simulink model "CRTsfun"  (Simulink 8.0)
settings: Solver=ode45  StartTime=0.0  StopTime=10.0  RelTol=1e-3
undefined symbols (not defined in the file or in its folder): vicrt_initcallback, vicrt_initmexcallback, vicrt_inputfile, vicrt_simulationmanager
(part 3 of 3)

== system CRTsfun/VI-CarRealTime/Output_Bus/adapter ==
  inputBus : Inport
  adaBCre : BusCreator  Inputs=24
  adaDemux : Demux  Outputs=24
  adaSel : Selector  InputPortWidth=24  IndexOptions=Select all  Indices=[1 3]  OutputSizes=1
  outputBus : Outport
  wires:
  adaBCre/1 -> outputBus/1
  adaDemux/24 -> adaBCre/24  "aero_forces:yaw_torque"
  adaDemux/23 -> adaBCre/23  "aero_forces:vertical_velocity"
  adaDemux/22 -> adaBCre/22  "aero_forces:steer"
  adaDemux/21 -> adaBCre/21  "aero_forces:side_slip"
  adaDemux/20 -> adaBCre/20  "aero_forces:roll_torque"
  adaDemux/19 -> adaBCre/19  "aero_forces:roll"
  adaDemux/18 -> adaBCre/18  "aero_forces:rear_sideforce"
  adaDemux/17 -> adaBCre/17  "aero_forces:rear_downforce"
  adaDemux/16 -> adaBCre/16  "aero_forces:pitch"
  adaDemux/15 -> adaBCre/15  "aero_forces:longitudinal_velocity"
  adaDemux/14 -> adaBCre/14  "aero_forces:lateral_velocity"
  adaDemux/13 -> adaBCre/13  "aero_forces:height_rear"
  adaDemux/12 -> adaBCre/12  "aero_forces:height_front"
  adaDemux/11 -> adaBCre/11  "aero_forces:height_auxiliary"
  adaDemux/10 -> adaBCre/10  "aero_forces:front_sideforce"
  adaDemux/9 -> adaBCre/9  "aero_forces:front_downforce"
  adaDemux/8 -> adaBCre/8  "aero_forces:drag_torque"
  adaDemux/7 -> adaBCre/7  "aero_forces:drag_force_rear"
  adaDemux/6 -> adaBCre/6  "aero_forces:drag_force_front"
  adaDemux/5 -> adaBCre/5  "aero_forces:drag_force"
  adaDemux/4 -> adaBCre/4  "aero_forces:drag_arm"
  adaDemux/3 -> adaBCre/3  "aero_forces:center_sideforce"
  adaDemux/2 -> adaBCre/2  "aero_forces:center_downforce"
  adaDemux/1 -> adaBCre/1  "aero_forces:aero_balance"
  adaSel/1 -> adaDemux/1
  inputBus/1 -> adaSel/1

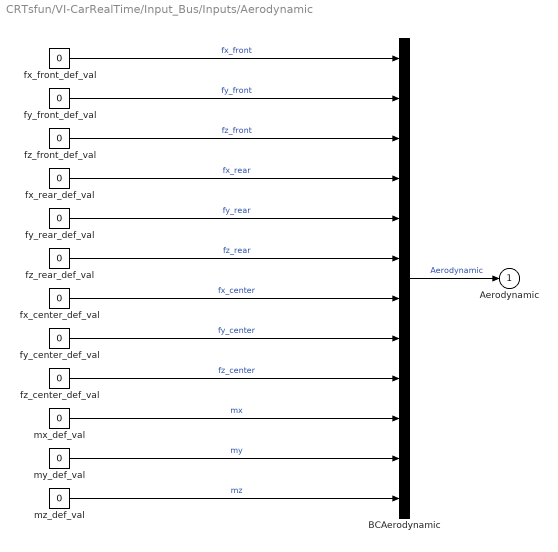
== system CRTsfun/VI-CarRealTime/Input_Bus/Inputs/Aerodynamic ==
  BCAerodynamic : BusCreator  Inputs=12
  fx_center_def_val : Constant  Value=0
  fx_front_def_val : Constant  Value=0
  fx_rear_def_val : Constant  Value=0
  fy_center_def_val : Constant  Value=0
  fy_front_def_val : Constant  Value=0
  fy_rear_def_val : Constant  Value=0
  fz_center_def_val : Constant  Value=0
  fz_front_def_val : Constant  Value=0
  fz_rear_def_val : Constant  Value=0
  mx_def_val : Constant  Value=0
  my_def_val : Constant  Value=0
  mz_def_val : Constant  Value=0
  Aerodynamic : Outport
  wires:
  mz_def_val/1 -> BCAerodynamic/12  "mz"
  my_def_val/1 -> BCAerodynamic/11  "my"
  mx_def_val/1 -> BCAerodynamic/10  "mx"
  fz_center_def_val/1 -> BCAerodynamic/9  "fz_center"
  fy_center_def_val/1 -> BCAerodynamic/8  "fy_center"
  fx_center_def_val/1 -> BCAerodynamic/7  "fx_center"
  fz_rear_def_val/1 -> BCAerodynamic/6  "fz_rear"
  fy_rear_def_val/1 -> BCAerodynamic/5  "fy_rear"
  fx_rear_def_val/1 -> BCAerodynamic/4  "fx_rear"
  fz_front_def_val/1 -> BCAerodynamic/3  "fz_front"
  fy_front_def_val/1 -> BCAerodynamic/2  "fy_front"
  fx_front_def_val/1 -> BCAerodynamic/1  "fx_front"
  BCAerodynamic/1 -> Aerodynamic/1  "Aerodynamic"

== system CRTsfun/VI-CarRealTime/Input_Bus/Inputs/Antiroll_Bar ==
  BCAntiroll_Bar : BusCreator  Inputs=2
  activity_flag : Subsystem
  force : Subsystem
  Antiroll_Bar : Outport
  wires:
  force/1(force) -> BCAntiroll_Bar/2  "force"
  activity_flag/1(activity_flag) -> BCAntiroll_Bar/1  "activity_flag"
  BCAntiroll_Bar/1 -> Antiroll_Bar/1  "Antiroll_Bar"

== system CRTsfun/VI-CarRealTime/Input_Bus/Inputs/Auxiliary_vertical ==
  BCAuxiliary_vertical : BusCreator  Inputs=2
  activity_flag : Subsystem
  force : Subsystem
  Auxiliary_vertical : Outport
  wires:
  activity_flag/1(activity_flag) -> BCAuxiliary_vertical/2  "activity_flag"
  force/1(force) -> BCAuxiliary_vertical/1  "force"
  BCAuxiliary_vertical/1 -> Auxiliary_vertical/1  "Auxiliary_vertical"

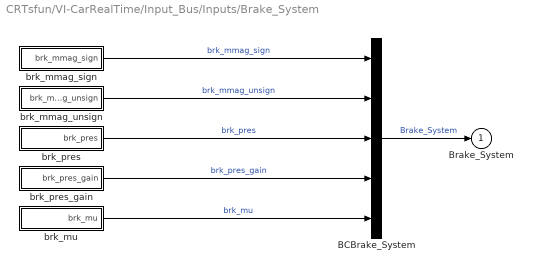
== system CRTsfun/VI-CarRealTime/Input_Bus/Inputs/Brake_System ==
  BCBrake_System : BusCreator  Inputs=5
  brk_mmag_sign : Subsystem
  brk_mmag_unsign : Subsystem
  brk_mu : Subsystem
  brk_pres : Subsystem
  brk_pres_gain : Subsystem
  Brake_System : Outport
  wires:
  brk_mu/1(brk_mu) -> BCBrake_System/5  "brk_mu"
  brk_pres_gain/1(brk_pres_gain) -> BCBrake_System/4  "brk_pres_gain"
  brk_pres/1(brk_pres) -> BCBrake_System/3  "brk_pres"
  brk_mmag_unsign/1(brk_mmag_unsign) -> BCBrake_System/2  "brk_mmag_unsign"
  brk_mmag_sign/1(brk_mmag_sign) -> BCBrake_System/1  "brk_mmag_sign"
  BCBrake_System/1 -> Brake_System/1  "Brake_System"

== system CRTsfun/VI-CarRealTime/Input_Bus/Inputs/Brake_System_General ==
  BCBrake_System_General : BusCreator  Inputs=2
  brk_bias_front_def_val : Constant  Value=0
  brk_mast_cyl_pres_def_val : Constant  Value=0
  Brake_System_General : Outport
  wires:
  brk_bias_front_def_val/1 -> BCBrake_System_General/2  "brk_bias_front"
  brk_mast_cyl_pres_def_val/1 -> BCBrake_System_General/1  "brk_mast_cyl_pres"
  BCBrake_System_General/1 -> Brake_System_General/1  "Brake_System_General"

== system CRTsfun/VI-CarRealTime/Input_Bus/Inputs/Clutch ==
  BCClutch : BusCreator  Inputs=2
  clutch_slip_angle_def_val : Constant  Value=0
  clutch_trq_def_val : Constant  Value=0
  Clutch : Outport
  wires:
  clutch_slip_angle_def_val/1 -> BCClutch/2  "clutch_slip_angle"
  clutch_trq_def_val/1 -> BCClutch/1  "clutch_trq"
  BCClutch/1 -> Clutch/1  "Clutch"

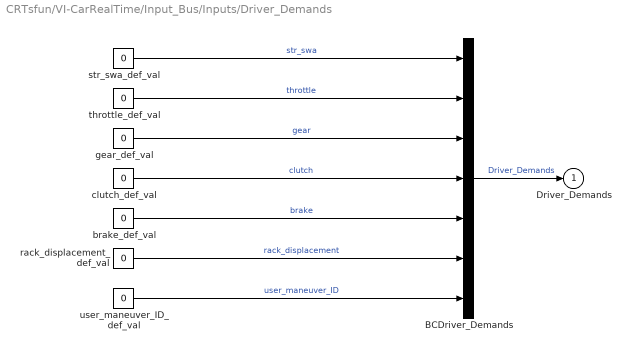
== system CRTsfun/VI-CarRealTime/Input_Bus/Inputs/Driver_Demands ==
  BCDriver_Demands : BusCreator  Inputs=7
  brake_def_val : Constant  Value=0
  clutch_def_val : Constant  Value=0
  gear_def_val : Constant  Value=0
  rack_displacement_def_val : Constant  Value=0
  str_swa_def_val : Constant  Value=0
  throttle_def_val : Constant  Value=0
  user_maneuver_ID_def_val : Constant  Value=0
  Driver_Demands : Outport
  wires:
  user_maneuver_ID_def_val/1 -> BCDriver_Demands/7  "user_maneuver_ID"
  rack_displacement_def_val/1 -> BCDriver_Demands/6  "rack_displacement"
  brake_def_val/1 -> BCDriver_Demands/5  "brake"
  clutch_def_val/1 -> BCDriver_Demands/4  "clutch"
  gear_def_val/1 -> BCDriver_Demands/3  "gear"
  throttle_def_val/1 -> BCDriver_Demands/2  "throttle"
  str_swa_def_val/1 -> BCDriver_Demands/1  "str_swa"
  BCDriver_Demands/1 -> Driver_Demands/1  "Driver_Demands"

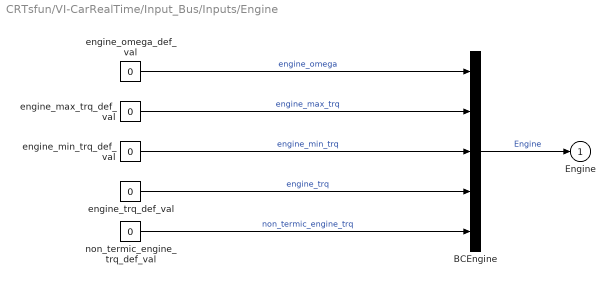
== system CRTsfun/VI-CarRealTime/Input_Bus/Inputs/Engine ==
  BCEngine : BusCreator  Inputs=5
  engine_max_trq_def_val : Constant  Value=0
  engine_min_trq_def_val : Constant  Value=0
  engine_omega_def_val : Constant  Value=0
  engine_trq_def_val : Constant  Value=0
  non_termic_engine_trq_def_val : Constant  Value=0
  Engine : Outport
  wires:
  non_termic_engine_trq_def_val/1 -> BCEngine/5  "non_termic_engine_trq"
  engine_trq_def_val/1 -> BCEngine/4  "engine_trq"
  engine_min_trq_def_val/1 -> BCEngine/3  "engine_min_trq"
  engine_max_trq_def_val/1 -> BCEngine/2  "engine_max_trq"
  engine_omega_def_val/1 -> BCEngine/1  "engine_omega"
  BCEngine/1 -> Engine/1  "Engine"

== system CRTsfun/VI-CarRealTime/Input_Bus/Inputs/Ext_Body ==
  BCExt_Body : BusCreator  Inputs=2
  force : Subsystem
  moment : Subsystem
  Ext_Body : Outport
  wires:
  moment/1(moment) -> BCExt_Body/2  "moment"
  force/1(force) -> BCExt_Body/1  "force"
  BCExt_Body/1 -> Ext_Body/1  "Ext_Body"

== system CRTsfun/VI-CarRealTime/Input_Bus/Inputs/Ext_Ground ==
  BCExt_Ground : BusCreator  Inputs=2
  force : Subsystem
  moment : Subsystem
  Ext_Ground : Outport
  wires:
  moment/1(moment) -> BCExt_Ground/2  "moment"
  force/1(force) -> BCExt_Ground/1  "force"
  BCExt_Ground/1 -> Ext_Ground/1  "Ext_Ground"

== system CRTsfun/VI-CarRealTime/Input_Bus/Inputs/Ext_Tracking ==
  BCExt_Tracking : BusCreator  Inputs=2
  force : Subsystem
  moment : Subsystem
  Ext_Tracking : Outport
  wires:
  moment/1(moment) -> BCExt_Tracking/2  "moment"
  force/1(force) -> BCExt_Tracking/1  "force"
  BCExt_Tracking/1 -> Ext_Tracking/1  "Ext_Tracking"

== system CRTsfun/VI-CarRealTime/Input_Bus/Inputs/Friction ==
  BCFriction : BusCreator  Inputs=1
  tire_mu : Subsystem
  Friction : Outport
  wires:
  tire_mu/1(tire_mu) -> BCFriction/1  "tire_mu"
  BCFriction/1 -> Friction/1  "Friction"

== system CRTsfun/VI-CarRealTime/Input_Bus/Inputs/GearBox ==
  BCGearBox : BusCreator  Inputs=1
  transmission_ratio_def_val : Constant  Value=0
  GearBox : Outport
  wires:
  transmission_ratio_def_val/1 -> BCGearBox/1  "transmission_ratio"
  BCGearBox/1 -> GearBox/1  "GearBox"

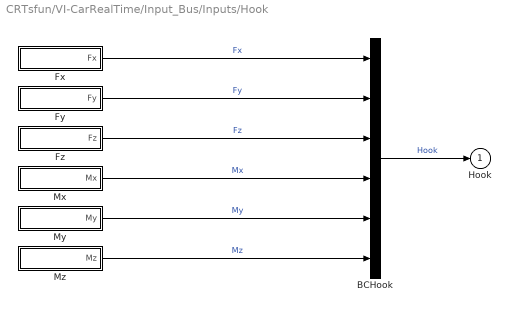
== system CRTsfun/VI-CarRealTime/Input_Bus/Inputs/Hook ==
  BCHook : BusCreator  Inputs=6
  Fx : Subsystem
  Fy : Subsystem
  Fz : Subsystem
  Mx : Subsystem
  My : Subsystem
  Mz : Subsystem
  Hook : Outport
  wires:
  Mz/1(Mz) -> BCHook/6  "Mz"
  My/1(My) -> BCHook/5  "My"
  Mx/1(Mx) -> BCHook/4  "Mx"
  Fz/1(Fz) -> BCHook/3  "Fz"
  Fy/1(Fy) -> BCHook/2  "Fy"
  Fx/1(Fx) -> BCHook/1  "Fx"
  BCHook/1 -> Hook/1  "Hook"

== system CRTsfun/VI-CarRealTime/Input_Bus/Inputs/Irregularity ==
  BCIrregularity : BusCreator  Inputs=1
  road : Subsystem
  Irregularity : Outport
  wires:
  road/1(road) -> BCIrregularity/1  "road"
  BCIrregularity/1 -> Irregularity/1  "Irregularity"

== system CRTsfun/VI-CarRealTime/Input_Bus/Inputs/Main_Bumpstop ==
  BCMain_Bumpstop : BusCreator  Inputs=2
  activity_flag : Subsystem
  force : Subsystem
  Main_Bumpstop : Outport
  wires:
  activity_flag/1(activity_flag) -> BCMain_Bumpstop/2  "activity_flag"
  force/1(force) -> BCMain_Bumpstop/1  "force"
  BCMain_Bumpstop/1 -> Main_Bumpstop/1  "Main_Bumpstop"

== system CRTsfun/VI-CarRealTime/Input_Bus/Inputs/Main_Damper ==
  BCMain_Damper : BusCreator  Inputs=2
  activity_flag : Subsystem
  force : Subsystem
  Main_Damper : Outport
  wires:
  activity_flag/1(activity_flag) -> BCMain_Damper/2  "activity_flag"
  force/1(force) -> BCMain_Damper/1  "force"
  BCMain_Damper/1 -> Main_Damper/1  "Main_Damper"

== system CRTsfun/VI-CarRealTime/Input_Bus/Inputs/Main_Reboundstop ==
  BCMain_Reboundstop : BusCreator  Inputs=2
  activity_flag : Subsystem
  force : Subsystem
  Main_Reboundstop : Outport
  wires:
  activity_flag/1(activity_flag) -> BCMain_Reboundstop/2  "activity_flag"
  force/1(force) -> BCMain_Reboundstop/1  "force"
  BCMain_Reboundstop/1 -> Main_Reboundstop/1  "Main_Reboundstop"

== system CRTsfun/VI-CarRealTime/Input_Bus/Inputs/Main_Spring ==
  BCMain_Spring : BusCreator  Inputs=2
  activity_flag : Subsystem
  force : Subsystem
  Main_Spring : Outport
  wires:
  activity_flag/1(activity_flag) -> BCMain_Spring/2  "activity_flag"
  force/1(force) -> BCMain_Spring/1  "force"
  BCMain_Spring/1 -> Main_Spring/1  "Main_Spring"

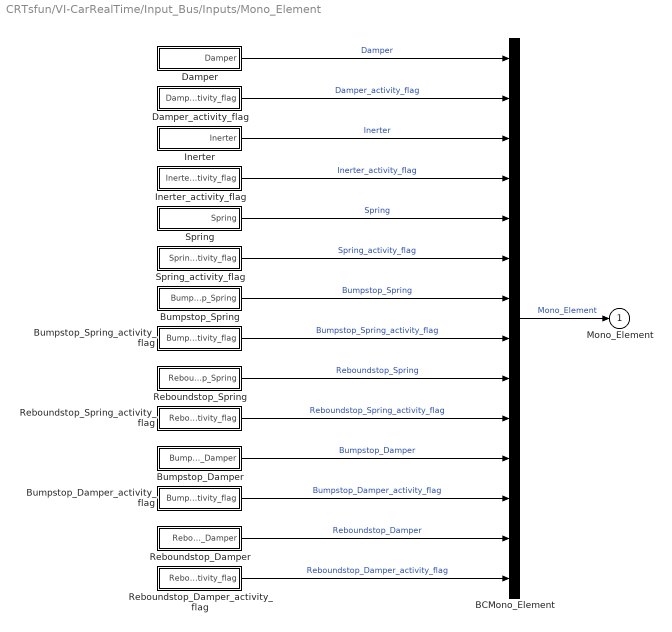
== system CRTsfun/VI-CarRealTime/Input_Bus/Inputs/Mono_Element ==
  BCMono_Element : BusCreator  Inputs=14
  Bumpstop_Damper : Subsystem
  Bumpstop_Damper_activity_flag : Subsystem
  Bumpstop_Spring : Subsystem
  Bumpstop_Spring_activity_flag : Subsystem
  Damper : Subsystem
  Damper_activity_flag : Subsystem
  Inerter : Subsystem
  Inerter_activity_flag : Subsystem
  Reboundstop_Damper : Subsystem
  Reboundstop_Damper_activity_flag : Subsystem
  Reboundstop_Spring : Subsystem
  Reboundstop_Spring_activity_flag : Subsystem
  Spring : Subsystem
  Spring_activity_flag : Subsystem
  Mono_Element : Outport
  wires:
  Reboundstop_Damper_activity_flag/1(Reboundstop_Damper_activity_flag) -> BCMono_Element/14  "Reboundstop_Damper_activity_flag"
  Reboundstop_Damper/1(Reboundstop_Damper) -> BCMono_Element/13  "Reboundstop_Damper"
  Bumpstop_Damper_activity_flag/1(Bumpstop_Damper_activity_flag) -> BCMono_Element/12  "Bumpstop_Damper_activity_flag"
  Bumpstop_Damper/1(Bumpstop_Damper) -> BCMono_Element/11  "Bumpstop_Damper"
  Reboundstop_Spring_activity_flag/1(Reboundstop_Spring_activity_flag) -> BCMono_Element/10  "Reboundstop_Spring_activity_flag"
  Reboundstop_Spring/1(Reboundstop_Spring) -> BCMono_Element/9  "Reboundstop_Spring"
  Bumpstop_Spring_activity_flag/1(Bumpstop_Spring_activity_flag) -> BCMono_Element/8  "Bumpstop_Spring_activity_flag"
  Bumpstop_Spring/1(Bumpstop_Spring) -> BCMono_Element/7  "Bumpstop_Spring"
  Spring_activity_flag/1(Spring_activity_flag) -> BCMono_Element/6  "Spring_activity_flag"
  Spring/1(Spring) -> BCMono_Element/5  "Spring"
  Inerter_activity_flag/1(Inerter_activity_flag) -> BCMono_Element/4  "Inerter_activity_flag"
  Inerter/1(Inerter) -> BCMono_Element/3  "Inerter"
  Damper_activity_flag/1(Damper_activity_flag) -> BCMono_Element/2  "Damper_activity_flag"
  Damper/1(Damper) -> BCMono_Element/1  "Damper"
  BCMono_Element/1 -> Mono_Element/1  "Mono_Element"

== system CRTsfun/VI-CarRealTime/Input_Bus/Inputs/Rear_Steering_Actuator_disp ==
  BCRear_Steering_Actuator_disp : BusCreator  Inputs=1
  str_swa : Subsystem
  Rear_Steering_Actuator_disp : Outport
  wires:
  str_swa/1(str_swa) -> BCRear_Steering_Actuator_disp/1  "str_swa"
  BCRear_Steering_Actuator_disp/1 -> Rear_Steering_Actuator_disp/1  "Rear_Steering_Actuator_disp"

== system CRTsfun/VI-CarRealTime/Input_Bus/Inputs/Steering ==
  BCSteering : BusCreator  Inputs=1
  steer_at_spindle : Subsystem
  Steering : Outport
  wires:
  steer_at_spindle/1(steer_at_spindle) -> BCSteering/1  "steer_at_spindle"
  BCSteering/1 -> Steering/1  "Steering"

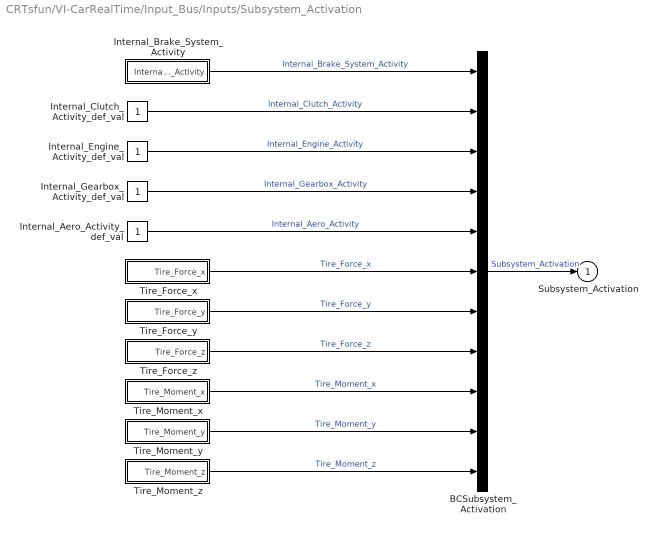
== system CRTsfun/VI-CarRealTime/Input_Bus/Inputs/Subsystem_Activation ==
  BCSubsystem_Activation : BusCreator  Inputs=11
  Internal_Aero_Activity_def_val : Constant
  Internal_Brake_System_Activity : Subsystem
  Internal_Clutch_Activity_def_val : Constant
  Internal_Engine_Activity_def_val : Constant
  Internal_Gearbox_Activity_def_val : Constant
  Tire_Force_x : Subsystem
  Tire_Force_y : Subsystem
  Tire_Force_z : Subsystem
  Tire_Moment_x : Subsystem
  Tire_Moment_y : Subsystem
  Tire_Moment_z : Subsystem
  Subsystem_Activation : Outport
  wires:
  Tire_Moment_z/1(Tire_Moment_z) -> BCSubsystem_Activation/11  "Tire_Moment_z"
  Tire_Moment_y/1(Tire_Moment_y) -> BCSubsystem_Activation/10  "Tire_Moment_y"
  Tire_Moment_x/1(Tire_Moment_x) -> BCSubsystem_Activation/9  "Tire_Moment_x"
  Tire_Force_z/1(Tire_Force_z) -> BCSubsystem_Activation/8  "Tire_Force_z"
  Tire_Force_y/1(Tire_Force_y) -> BCSubsystem_Activation/7  "Tire_Force_y"
  Tire_Force_x/1(Tire_Force_x) -> BCSubsystem_Activation/6  "Tire_Force_x"
  Internal_Aero_Activity_def_val/1 -> BCSubsystem_Activation/5  "Internal_Aero_Activity"
  Internal_Gearbox_Activity_def_val/1 -> BCSubsystem_Activation/4  "Internal_Gearbox_Activity"
  Internal_Engine_Activity_def_val/1 -> BCSubsystem_Activation/3  "Internal_Engine_Activity"
  Internal_Clutch_Activity_def_val/1 -> BCSubsystem_Activation/2  "Internal_Clutch_Activity"
  Internal_Brake_System_Activity/1(Internal_Brake_System_Activity) -> BCSubsystem_Activation/1  "Internal_Brake_System_Activity"
  BCSubsystem_Activation/1 -> Subsystem_Activation/1  "Subsystem_Activation"

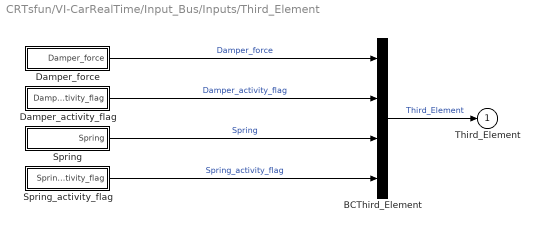
== system CRTsfun/VI-CarRealTime/Input_Bus/Inputs/Third_Element ==
  BCThird_Element : BusCreator
  Damper_activity_flag : Subsystem
  Damper_force : Subsystem
  Spring : Subsystem
  Spring_activity_flag : Subsystem
  Third_Element : Outport
  wires:
  Spring_activity_flag/1(Spring_activity_flag) -> BCThird_Element/4  "Spring_activity_flag"
  Spring/1(Spring) -> BCThird_Element/3  "Spring"
  Damper_activity_flag/1(Damper_activity_flag) -> BCThird_Element/2  "Damper_activity_flag"
  Damper_force/1(Damper_force) -> BCThird_Element/1  "Damper_force"
  BCThird_Element/1 -> Third_Element/1  "Third_Element"

== system CRTsfun/VI-CarRealTime/Input_Bus/Inputs/Tire_Force ==
  BCTire_Force : BusCreator  Inputs=3
  Fx : Subsystem
  Fy : Subsystem
  Fz : Subsystem
  Tire_Force : Outport
  wires:
  Fz/1(Fz) -> BCTire_Force/3  "Fz"
  Fy/1(Fy) -> BCTire_Force/2  "Fy"
  Fx/1(Fx) -> BCTire_Force/1  "Fx"
  BCTire_Force/1 -> Tire_Force/1  "Tire_Force"

== system CRTsfun/VI-CarRealTime/Input_Bus/Inputs/Tire_Moment ==
  BCTire_Moment : BusCreator  Inputs=3
  Mx : Subsystem
  My : Subsystem
  Mz : Subsystem
  Tire_Moment : Outport
  wires:
  Mz/1(Mz) -> BCTire_Moment/3  "Mz"
  My/1(My) -> BCTire_Moment/2  "My"
  Mx/1(Mx) -> BCTire_Moment/1  "Mx"
  BCTire_Moment/1 -> Tire_Moment/1  "Tire_Moment"

== system CRTsfun/VI-CarRealTime/Input_Bus/Inputs/Wheel_driving ==
  BCWheel_driving : BusCreator  Inputs=1
  moment : Subsystem
  Wheel_driving : Outport
  wires:
  moment/1(moment) -> BCWheel_driving/1  "moment"
  BCWheel_driving/1 -> Wheel_driving/1  "Wheel_driving"

== system CRTsfun/VI-CarRealTime/Input_Bus/Inputs/Antiroll_Bar/activity_flag ==
  BCactivity_flag : BusCreator  Inputs=2
  front_def_val : Constant
  rear_def_val : Constant
  activity_flag : Outport
  wires:
  rear_def_val/1 -> BCactivity_flag/2  "rear"
  front_def_val/1 -> BCactivity_flag/1  "front"
  BCactivity_flag/1 -> activity_flag/1  "activity_flag"

== system CRTsfun/VI-CarRealTime/Input_Bus/Inputs/Antiroll_Bar/force ==
  BCforce : BusCreator  Inputs=2
  front_def_val : Constant  Value=0
  rear_def_val : Constant  Value=0
  force : Outport
  wires:
  rear_def_val/1 -> BCforce/2  "rear"
  front_def_val/1 -> BCforce/1  "front"
  BCforce/1 -> force/1  "force"

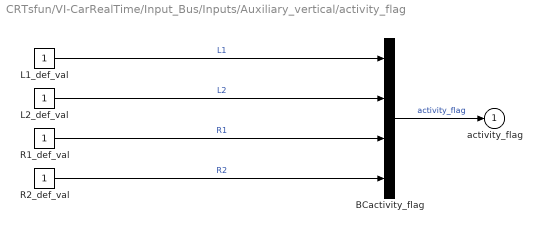
== system CRTsfun/VI-CarRealTime/Input_Bus/Inputs/Auxiliary_vertical/activity_flag ==
  BCactivity_flag : BusCreator
  L1_def_val : Constant
  L2_def_val : Constant
  R1_def_val : Constant
  R2_def_val : Constant
  activity_flag : Outport
  wires:
  R2_def_val/1 -> BCactivity_flag/4  "R2"
  R1_def_val/1 -> BCactivity_flag/3  "R1"
  L2_def_val/1 -> BCactivity_flag/2  "L2"
  L1_def_val/1 -> BCactivity_flag/1  "L1"
  BCactivity_flag/1 -> activity_flag/1  "activity_flag"

== system CRTsfun/VI-CarRealTime/Input_Bus/Inputs/Auxiliary_vertical/force ==
  BCforce : BusCreator
  L1_def_val : Constant  Value=0
  L2_def_val : Constant  Value=0
  R1_def_val : Constant  Value=0
  R2_def_val : Constant  Value=0
  force : Outport
  wires:
  R2_def_val/1 -> BCforce/4  "R2"
  R1_def_val/1 -> BCforce/3  "R1"
  L2_def_val/1 -> BCforce/2  "L2"
  L1_def_val/1 -> BCforce/1  "L1"
  BCforce/1 -> force/1  "force"

== system CRTsfun/VI-CarRealTime/Input_Bus/Inputs/Brake_System/brk_mmag_sign ==
  BCbrk_mmag_sign : BusCreator
  L1_def_val : Constant  Value=0
  L2_def_val : Constant  Value=0
  R1_def_val : Constant  Value=0
  R2_def_val : Constant  Value=0
  brk_mmag_sign : Outport
  wires:
  R2_def_val/1 -> BCbrk_mmag_sign/4  "R2"
  R1_def_val/1 -> BCbrk_mmag_sign/3  "R1"
  L2_def_val/1 -> BCbrk_mmag_sign/2  "L2"
  L1_def_val/1 -> BCbrk_mmag_sign/1  "L1"
  BCbrk_mmag_sign/1 -> brk_mmag_sign/1  "brk_mmag_sign"

== system CRTsfun/VI-CarRealTime/Input_Bus/Inputs/Brake_System/brk_mmag_unsign ==
  BCbrk_mmag_unsign : BusCreator
  L1_def_val : Constant  Value=0
  L2_def_val : Constant  Value=0
  R1_def_val : Constant  Value=0
  R2_def_val : Constant  Value=0
  brk_mmag_unsign : Outport
  wires:
  R2_def_val/1 -> BCbrk_mmag_unsign/4  "R2"
  R1_def_val/1 -> BCbrk_mmag_unsign/3  "R1"
  L2_def_val/1 -> BCbrk_mmag_unsign/2  "L2"
  L1_def_val/1 -> BCbrk_mmag_unsign/1  "L1"
  BCbrk_mmag_unsign/1 -> brk_mmag_unsign/1  "brk_mmag_unsign"

== system CRTsfun/VI-CarRealTime/Input_Bus/Inputs/Brake_System/brk_mu ==
  BCbrk_mu : BusCreator
  L1_def_val : Constant  Value=0
  L2_def_val : Constant  Value=0
  R1_def_val : Constant  Value=0
  R2_def_val : Constant  Value=0
  brk_mu : Outport
  wires:
  R2_def_val/1 -> BCbrk_mu/4  "R2"
  R1_def_val/1 -> BCbrk_mu/3  "R1"
  L2_def_val/1 -> BCbrk_mu/2  "L2"
  L1_def_val/1 -> BCbrk_mu/1  "L1"
  BCbrk_mu/1 -> brk_mu/1  "brk_mu"

== system CRTsfun/VI-CarRealTime/Input_Bus/Inputs/Brake_System/brk_pres ==
  BCbrk_pres : BusCreator
  L1_def_val : Constant  Value=0
  L2_def_val : Constant  Value=0
  R1_def_val : Constant  Value=0
  R2_def_val : Constant  Value=0
  brk_pres : Outport
  wires:
  R2_def_val/1 -> BCbrk_pres/4  "R2"
  R1_def_val/1 -> BCbrk_pres/3  "R1"
  L2_def_val/1 -> BCbrk_pres/2  "L2"
  L1_def_val/1 -> BCbrk_pres/1  "L1"
  BCbrk_pres/1 -> brk_pres/1  "brk_pres"

== system CRTsfun/VI-CarRealTime/Input_Bus/Inputs/Brake_System/brk_pres_gain ==
  BCbrk_pres_gain : BusCreator
  L1_def_val : Constant
  L2_def_val : Constant
  R1_def_val : Constant
  R2_def_val : Constant
  brk_pres_gain : Outport
  wires:
  R2_def_val/1 -> BCbrk_pres_gain/4  "R2"
  R1_def_val/1 -> BCbrk_pres_gain/3  "R1"
  L2_def_val/1 -> BCbrk_pres_gain/2  "L2"
  L1_def_val/1 -> BCbrk_pres_gain/1  "L1"
  BCbrk_pres_gain/1 -> brk_pres_gain/1  "brk_pres_gain"

== system CRTsfun/VI-CarRealTime/Input_Bus/Inputs/Ext_Body/force ==
  BCforce : BusCreator  Inputs=3
  X_def_val : Constant  Value=0
  Y_def_val : Constant  Value=0
  Z_def_val : Constant  Value=0
  force : Outport
  wires:
  Z_def_val/1 -> BCforce/3  "Z"
  Y_def_val/1 -> BCforce/2  "Y"
  X_def_val/1 -> BCforce/1  "X"
  BCforce/1 -> force/1  "force"

== system CRTsfun/VI-CarRealTime/Input_Bus/Inputs/Ext_Body/moment ==
  BCmoment : BusCreator  Inputs=3
  X_def_val : Constant  Value=0
  Y_def_val : Constant  Value=0
  Z_def_val : Constant  Value=0
  moment : Outport
  wires:
  Z_def_val/1 -> BCmoment/3  "Z"
  Y_def_val/1 -> BCmoment/2  "Y"
  X_def_val/1 -> BCmoment/1  "X"
  BCmoment/1 -> moment/1  "moment"

== system CRTsfun/VI-CarRealTime/Input_Bus/Inputs/Ext_Ground/force ==
  BCforce : BusCreator  Inputs=3
  X_def_val : Constant  Value=0
  Y_def_val : Constant  Value=0
  Z_def_val : Constant  Value=0
  force : Outport
  wires:
  Z_def_val/1 -> BCforce/3  "Z"
  Y_def_val/1 -> BCforce/2  "Y"
  X_def_val/1 -> BCforce/1  "X"
  BCforce/1 -> force/1  "force"

== system CRTsfun/VI-CarRealTime/Input_Bus/Inputs/Ext_Ground/moment ==
  BCmoment : BusCreator  Inputs=3
  X_def_val : Constant  Value=0
  Y_def_val : Constant  Value=0
  Z_def_val : Constant  Value=0
  moment : Outport
  wires:
  Z_def_val/1 -> BCmoment/3  "Z"
  Y_def_val/1 -> BCmoment/2  "Y"
  X_def_val/1 -> BCmoment/1  "X"
  BCmoment/1 -> moment/1  "moment"

== system CRTsfun/VI-CarRealTime/Input_Bus/Inputs/Ext_Tracking/force ==
  BCforce : BusCreator  Inputs=2
  X_def_val : Constant  Value=0
  Y_def_val : Constant  Value=0
  force : Outport
  wires:
  Y_def_val/1 -> BCforce/2  "Y"
  X_def_val/1 -> BCforce/1  "X"
  BCforce/1 -> force/1  "force"

== system CRTsfun/VI-CarRealTime/Input_Bus/Inputs/Ext_Tracking/moment ==
  BCmoment : BusCreator  Inputs=2
  X_def_val : Constant  Value=0
  Y_def_val : Constant  Value=0
  moment : Outport
  wires:
  Y_def_val/1 -> BCmoment/2  "Y"
  X_def_val/1 -> BCmoment/1  "X"
  BCmoment/1 -> moment/1  "moment"

== system CRTsfun/VI-CarRealTime/Input_Bus/Inputs/Friction/tire_mu ==
  BCtire_mu : BusCreator
  L1_def_val : Constant  Value=0
  L2_def_val : Constant  Value=0
  R1_def_val : Constant  Value=0
  R2_def_val : Constant  Value=0
  tire_mu : Outport
  wires:
  R2_def_val/1 -> BCtire_mu/4  "R2"
  R1_def_val/1 -> BCtire_mu/3  "R1"
  L2_def_val/1 -> BCtire_mu/2  "L2"
  L1_def_val/1 -> BCtire_mu/1  "L1"
  BCtire_mu/1 -> tire_mu/1  "tire_mu"

== system CRTsfun/VI-CarRealTime/Input_Bus/Inputs/Hook/Fx ==
  BCFx : BusCreator  Inputs=1
  rear_def_val : Constant  Value=0
  Fx : Outport
  wires:
  rear_def_val/1 -> BCFx/1  "rear"
  BCFx/1 -> Fx/1  "Fx"

== system CRTsfun/VI-CarRealTime/Input_Bus/Inputs/Hook/Fy ==
  BCFy : BusCreator  Inputs=1
  rear_def_val : Constant  Value=0
  Fy : Outport
  wires:
  rear_def_val/1 -> BCFy/1  "rear"
  BCFy/1 -> Fy/1  "Fy"

== system CRTsfun/VI-CarRealTime/Input_Bus/Inputs/Hook/Fz ==
  BCFz : BusCreator  Inputs=1
  rear_def_val : Constant  Value=0
  Fz : Outport
  wires:
  rear_def_val/1 -> BCFz/1  "rear"
  BCFz/1 -> Fz/1  "Fz"

== system CRTsfun/VI-CarRealTime/Input_Bus/Inputs/Hook/Mx ==
  BCMx : BusCreator  Inputs=1
  rear_def_val : Constant  Value=0
  Mx : Outport
  wires:
  rear_def_val/1 -> BCMx/1  "rear"
  BCMx/1 -> Mx/1  "Mx"

== system CRTsfun/VI-CarRealTime/Input_Bus/Inputs/Hook/My ==
  BCMy : BusCreator  Inputs=1
  rear_def_val : Constant  Value=0
  My : Outport
  wires:
  rear_def_val/1 -> BCMy/1  "rear"
  BCMy/1 -> My/1  "My"

== system CRTsfun/VI-CarRealTime/Input_Bus/Inputs/Hook/Mz ==
  BCMz : BusCreator  Inputs=1
  rear_def_val : Constant  Value=0
  Mz : Outport
  wires:
  rear_def_val/1 -> BCMz/1  "rear"
  BCMz/1 -> Mz/1  "Mz"

== system CRTsfun/VI-CarRealTime/Input_Bus/Inputs/Irregularity/road ==
  BCroad : BusCreator
  L1_def_val : Constant  Value=0
  L2_def_val : Constant  Value=0
  R1_def_val : Constant  Value=0
  R2_def_val : Constant  Value=0
  road : Outport
  wires:
  R2_def_val/1 -> BCroad/4  "R2"
  R1_def_val/1 -> BCroad/3  "R1"
  L2_def_val/1 -> BCroad/2  "L2"
  L1_def_val/1 -> BCroad/1  "L1"
  BCroad/1 -> road/1  "road"

== system CRTsfun/VI-CarRealTime/Input_Bus/Inputs/Main_Bumpstop/activity_flag ==
  BCactivity_flag : BusCreator
  L1_def_val : Constant
  L2_def_val : Constant
  R1_def_val : Constant
  R2_def_val : Constant
  activity_flag : Outport
  wires:
  R2_def_val/1 -> BCactivity_flag/4  "R2"
  R1_def_val/1 -> BCactivity_flag/3  "R1"
  L2_def_val/1 -> BCactivity_flag/2  "L2"
  L1_def_val/1 -> BCactivity_flag/1  "L1"
  BCactivity_flag/1 -> activity_flag/1  "activity_flag"

== system CRTsfun/VI-CarRealTime/Input_Bus/Inputs/Main_Bumpstop/force ==
  BCforce : BusCreator
  L1_def_val : Constant  Value=0
  L2_def_val : Constant  Value=0
  R1_def_val : Constant  Value=0
  R2_def_val : Constant  Value=0
  force : Outport
  wires:
  R2_def_val/1 -> BCforce/4  "R2"
  R1_def_val/1 -> BCforce/3  "R1"
  L2_def_val/1 -> BCforce/2  "L2"
  L1_def_val/1 -> BCforce/1  "L1"
  BCforce/1 -> force/1  "force"

== system CRTsfun/VI-CarRealTime/Input_Bus/Inputs/Main_Damper/activity_flag ==
  BCactivity_flag : BusCreator
  L1_def_val : Constant
  L2_def_val : Constant
  R1_def_val : Constant
  R2_def_val : Constant
  activity_flag : Outport
  wires:
  R2_def_val/1 -> BCactivity_flag/4  "R2"
  R1_def_val/1 -> BCactivity_flag/3  "R1"
  L2_def_val/1 -> BCactivity_flag/2  "L2"
  L1_def_val/1 -> BCactivity_flag/1  "L1"
  BCactivity_flag/1 -> activity_flag/1  "activity_flag"

== system CRTsfun/VI-CarRealTime/Input_Bus/Inputs/Main_Damper/force ==
  BCforce : BusCreator
  L1_def_val : Constant  Value=0
  L2_def_val : Constant  Value=0
  R1_def_val : Constant  Value=0
  R2_def_val : Constant  Value=0
  force : Outport
  wires:
  R2_def_val/1 -> BCforce/4  "R2"
  R1_def_val/1 -> BCforce/3  "R1"
  L2_def_val/1 -> BCforce/2  "L2"
  L1_def_val/1 -> BCforce/1  "L1"
  BCforce/1 -> force/1  "force"

== system CRTsfun/VI-CarRealTime/Input_Bus/Inputs/Main_Reboundstop/activity_flag ==
  BCactivity_flag : BusCreator
  L1_def_val : Constant
  L2_def_val : Constant
  R1_def_val : Constant
  R2_def_val : Constant
  activity_flag : Outport
  wires:
  R2_def_val/1 -> BCactivity_flag/4  "R2"
  R1_def_val/1 -> BCactivity_flag/3  "R1"
  L2_def_val/1 -> BCactivity_flag/2  "L2"
  L1_def_val/1 -> BCactivity_flag/1  "L1"
  BCactivity_flag/1 -> activity_flag/1  "activity_flag"

== system CRTsfun/VI-CarRealTime/Input_Bus/Inputs/Main_Reboundstop/force ==
  BCforce : BusCreator
  L1_def_val : Constant  Value=0
  L2_def_val : Constant  Value=0
  R1_def_val : Constant  Value=0
  R2_def_val : Constant  Value=0
  force : Outport
  wires:
  R2_def_val/1 -> BCforce/4  "R2"
  R1_def_val/1 -> BCforce/3  "R1"
  L2_def_val/1 -> BCforce/2  "L2"
  L1_def_val/1 -> BCforce/1  "L1"
  BCforce/1 -> force/1  "force"

== system CRTsfun/VI-CarRealTime/Input_Bus/Inputs/Main_Spring/activity_flag ==
  BCactivity_flag : BusCreator
  L1_def_val : Constant
  L2_def_val : Constant
  R1_def_val : Constant
  R2_def_val : Constant
  activity_flag : Outport
  wires:
  R2_def_val/1 -> BCactivity_flag/4  "R2"
  R1_def_val/1 -> BCactivity_flag/3  "R1"
  L2_def_val/1 -> BCactivity_flag/2  "L2"
  L1_def_val/1 -> BCactivity_flag/1  "L1"
  BCactivity_flag/1 -> activity_flag/1  "activity_flag"

== system CRTsfun/VI-CarRealTime/Input_Bus/Inputs/Main_Spring/force ==
  BCforce : BusCreator
  L1_def_val : Constant  Value=0
  L2_def_val : Constant  Value=0
  R1_def_val : Constant  Value=0
  R2_def_val : Constant  Value=0
  force : Outport
  wires:
  R2_def_val/1 -> BCforce/4  "R2"
  R1_def_val/1 -> BCforce/3  "R1"
  L2_def_val/1 -> BCforce/2  "L2"
  L1_def_val/1 -> BCforce/1  "L1"
  BCforce/1 -> force/1  "force"

== system CRTsfun/VI-CarRealTime/Input_Bus/Inputs/Mono_Element/Bumpstop_Damper ==
  BCBumpstop_Damper : BusCreator  Inputs=2
  front_def_val : Constant  Value=0
  rear_def_val : Constant  Value=0
  Bumpstop_Damper : Outport
  wires:
  rear_def_val/1 -> BCBumpstop_Damper/2  "rear"
  front_def_val/1 -> BCBumpstop_Damper/1  "front"
  BCBumpstop_Damper/1 -> Bumpstop_Damper/1  "Bumpstop_Damper"

== system CRTsfun/VI-CarRealTime/Input_Bus/Inputs/Mono_Element/Bumpstop_Damper_activity_flag ==
  BCBumpstop_Damper_activity_flag : BusCreator  Inputs=2
  front_def_val : Constant
  rear_def_val : Constant
  Bumpstop_Damper_activity_flag : Outport
  wires:
  rear_def_val/1 -> BCBumpstop_Damper_activity_flag/2  "rear"
  front_def_val/1 -> BCBumpstop_Damper_activity_flag/1  "front"
  BCBumpstop_Damper_activity_flag/1 -> Bumpstop_Damper_activity_flag/1  "Bumpstop_Damper_activity_flag"

== system CRTsfun/VI-CarRealTime/Input_Bus/Inputs/Mono_Element/Bumpstop_Spring ==
  BCBumpstop_Spring : BusCreator  Inputs=2
  front_def_val : Constant  Value=0
  rear_def_val : Constant  Value=0
  Bumpstop_Spring : Outport
  wires:
  rear_def_val/1 -> BCBumpstop_Spring/2  "rear"
  front_def_val/1 -> BCBumpstop_Spring/1  "front"
  BCBumpstop_Spring/1 -> Bumpstop_Spring/1  "Bumpstop_Spring"

== system CRTsfun/VI-CarRealTime/Input_Bus/Inputs/Mono_Element/Bumpstop_Spring_activity_flag ==
  BCBumpstop_Spring_activity_flag : BusCreator  Inputs=2
  front_def_val : Constant
  rear_def_val : Constant
  Bumpstop_Spring_activity_flag : Outport
  wires:
  rear_def_val/1 -> BCBumpstop_Spring_activity_flag/2  "rear"
  front_def_val/1 -> BCBumpstop_Spring_activity_flag/1  "front"
  BCBumpstop_Spring_activity_flag/1 -> Bumpstop_Spring_activity_flag/1  "Bumpstop_Spring_activity_flag"

== system CRTsfun/VI-CarRealTime/Input_Bus/Inputs/Mono_Element/Damper ==
  BCDamper : BusCreator  Inputs=2
  front_def_val : Constant  Value=0
  rear_def_val : Constant  Value=0
  Damper : Outport
  wires:
  rear_def_val/1 -> BCDamper/2  "rear"
  front_def_val/1 -> BCDamper/1  "front"
  BCDamper/1 -> Damper/1  "Damper"

== system CRTsfun/VI-CarRealTime/Input_Bus/Inputs/Mono_Element/Damper_activity_flag ==
  BCDamper_activity_flag : BusCreator  Inputs=2
  front_def_val : Constant
  rear_def_val : Constant
  Damper_activity_flag : Outport
  wires:
  rear_def_val/1 -> BCDamper_activity_flag/2  "rear"
  front_def_val/1 -> BCDamper_activity_flag/1  "front"
  BCDamper_activity_flag/1 -> Damper_activity_flag/1  "Damper_activity_flag"

== system CRTsfun/VI-CarRealTime/Input_Bus/Inputs/Mono_Element/Inerter ==
  BCInerter : BusCreator  Inputs=2
  front_def_val : Constant  Value=0
  rear_def_val : Constant  Value=0
  Inerter : Outport
  wires:
  rear_def_val/1 -> BCInerter/2  "rear"
  front_def_val/1 -> BCInerter/1  "front"
  BCInerter/1 -> Inerter/1  "Inerter"

== system CRTsfun/VI-CarRealTime/Input_Bus/Inputs/Mono_Element/Inerter_activity_flag ==
  BCInerter_activity_flag : BusCreator  Inputs=2
  front_def_val : Constant
  rear_def_val : Constant
  Inerter_activity_flag : Outport
  wires:
  rear_def_val/1 -> BCInerter_activity_flag/2  "rear"
  front_def_val/1 -> BCInerter_activity_flag/1  "front"
  BCInerter_activity_flag/1 -> Inerter_activity_flag/1  "Inerter_activity_flag"

== system CRTsfun/VI-CarRealTime/Input_Bus/Inputs/Mono_Element/Reboundstop_Damper ==
  BCReboundstop_Damper : BusCreator  Inputs=2
  front_def_val : Constant  Value=0
  rear_def_val : Constant  Value=0
  Reboundstop_Damper : Outport
  wires:
  rear_def_val/1 -> BCReboundstop_Damper/2  "rear"
  front_def_val/1 -> BCReboundstop_Damper/1  "front"
  BCReboundstop_Damper/1 -> Reboundstop_Damper/1  "Reboundstop_Damper"

== system CRTsfun/VI-CarRealTime/Input_Bus/Inputs/Mono_Element/Reboundstop_Damper_activity_flag ==
  BCReboundstop_Damper_activity_flag : BusCreator  Inputs=2
  front_def_val : Constant
  rear_def_val : Constant
  Reboundstop_Damper_activity_flag : Outport
  wires:
  rear_def_val/1 -> BCReboundstop_Damper_activity_flag/2  "rear"
  front_def_val/1 -> BCReboundstop_Damper_activity_flag/1  "front"
  BCReboundstop_Damper_activity_flag/1 -> Reboundstop_Damper_activity_flag/1  "Reboundstop_Damper_activity_flag"

== system CRTsfun/VI-CarRealTime/Input_Bus/Inputs/Mono_Element/Reboundstop_Spring ==
  BCReboundstop_Spring : BusCreator  Inputs=2
  front_def_val : Constant  Value=0
  rear_def_val : Constant  Value=0
  Reboundstop_Spring : Outport
  wires:
  rear_def_val/1 -> BCReboundstop_Spring/2  "rear"
  front_def_val/1 -> BCReboundstop_Spring/1  "front"
  BCReboundstop_Spring/1 -> Reboundstop_Spring/1  "Reboundstop_Spring"

== system CRTsfun/VI-CarRealTime/Input_Bus/Inputs/Mono_Element/Reboundstop_Spring_activity_flag ==
  BCReboundstop_Spring_activity_flag : BusCreator  Inputs=2
  front_def_val : Constant
  rear_def_val : Constant
  Reboundstop_Spring_activity_flag : Outport
  wires:
  rear_def_val/1 -> BCReboundstop_Spring_activity_flag/2  "rear"
  front_def_val/1 -> BCReboundstop_Spring_activity_flag/1  "front"
  BCReboundstop_Spring_activity_flag/1 -> Reboundstop_Spring_activity_flag/1  "Reboundstop_Spring_activity_flag"

== system CRTsfun/VI-CarRealTime/Input_Bus/Inputs/Mono_Element/Spring ==
  BCSpring : BusCreator  Inputs=2
  front_def_val : Constant  Value=0
  rear_def_val : Constant  Value=0
  Spring : Outport
  wires:
  rear_def_val/1 -> BCSpring/2  "rear"
  front_def_val/1 -> BCSpring/1  "front"
  BCSpring/1 -> Spring/1  "Spring"

== system CRTsfun/VI-CarRealTime/Input_Bus/Inputs/Mono_Element/Spring_activity_flag ==
  BCSpring_activity_flag : BusCreator  Inputs=2
  front_def_val : Constant
  rear_def_val : Constant
  Spring_activity_flag : Outport
  wires:
  rear_def_val/1 -> BCSpring_activity_flag/2  "rear"
  front_def_val/1 -> BCSpring_activity_flag/1  "front"
  BCSpring_activity_flag/1 -> Spring_activity_flag/1  "Spring_activity_flag"

== system CRTsfun/VI-CarRealTime/Input_Bus/Inputs/Rear_Steering_Actuator_disp/str_swa ==
  BCstr_swa : BusCreator  Inputs=2
  left_def_val : Constant  Value=0
  right_def_val : Constant  Value=0
  str_swa : Outport
  wires:
  right_def_val/1 -> BCstr_swa/2  "right"
  left_def_val/1 -> BCstr_swa/1  "left"
  BCstr_swa/1 -> str_swa/1  "str_swa"

== system CRTsfun/VI-CarRealTime/Input_Bus/Inputs/Steering/steer_at_spindle ==
  BCsteer_at_spindle : BusCreator
  L1_def_val : Constant  Value=0
  L2_def_val : Constant  Value=0
  R1_def_val : Constant  Value=0
  R2_def_val : Constant  Value=0
  steer_at_spindle : Outport
  wires:
  R2_def_val/1 -> BCsteer_at_spindle/4  "R2"
  R1_def_val/1 -> BCsteer_at_spindle/3  "R1"
  L2_def_val/1 -> BCsteer_at_spindle/2  "L2"
  L1_def_val/1 -> BCsteer_at_spindle/1  "L1"
  BCsteer_at_spindle/1 -> steer_at_spindle/1  "steer_at_spindle"

== system CRTsfun/VI-CarRealTime/Input_Bus/Inputs/Subsystem_Activation/Internal_Brake_System_Activity ==
  BCInternal_Brake_System_Activity : BusCreator
  L1_def_val : Constant
  L2_def_val : Constant
  R1_def_val : Constant
  R2_def_val : Constant
  Internal_Brake_System_Activity : Outport
  wires:
  R2_def_val/1 -> BCInternal_Brake_System_Activity/4  "R2"
  R1_def_val/1 -> BCInternal_Brake_System_Activity/3  "R1"
  L2_def_val/1 -> BCInternal_Brake_System_Activity/2  "L2"
  L1_def_val/1 -> BCInternal_Brake_System_Activity/1  "L1"
  BCInternal_Brake_System_Activity/1 -> Internal_Brake_System_Activity/1  "Internal_Brake_System_Activity"

== system CRTsfun/VI-CarRealTime/Input_Bus/Inputs/Subsystem_Activation/Tire_Force_x ==
  BCTire_Force_x : BusCreator
  L1_def_val : Constant
  L2_def_val : Constant
  R1_def_val : Constant
  R2_def_val : Constant
  Tire_Force_x : Outport
  wires:
  R2_def_val/1 -> BCTire_Force_x/4  "R2"
  R1_def_val/1 -> BCTire_Force_x/3  "R1"
  L2_def_val/1 -> BCTire_Force_x/2  "L2"
  L1_def_val/1 -> BCTire_Force_x/1  "L1"
  BCTire_Force_x/1 -> Tire_Force_x/1  "Tire_Force_x"

== system CRTsfun/VI-CarRealTime/Input_Bus/Inputs/Subsystem_Activation/Tire_Force_y ==
  BCTire_Force_y : BusCreator
  L1_def_val : Constant
  L2_def_val : Constant
  R1_def_val : Constant
  R2_def_val : Constant
  Tire_Force_y : Outport
  wires:
  R2_def_val/1 -> BCTire_Force_y/4  "R2"
  R1_def_val/1 -> BCTire_Force_y/3  "R1"
  L2_def_val/1 -> BCTire_Force_y/2  "L2"
  L1_def_val/1 -> BCTire_Force_y/1  "L1"
  BCTire_Force_y/1 -> Tire_Force_y/1  "Tire_Force_y"

== system CRTsfun/VI-CarRealTime/Input_Bus/Inputs/Subsystem_Activation/Tire_Force_z ==
  BCTire_Force_z : BusCreator
  L1_def_val : Constant
  L2_def_val : Constant
  R1_def_val : Constant
  R2_def_val : Constant
  Tire_Force_z : Outport
  wires:
  R2_def_val/1 -> BCTire_Force_z/4  "R2"
  R1_def_val/1 -> BCTire_Force_z/3  "R1"
  L2_def_val/1 -> BCTire_Force_z/2  "L2"
  L1_def_val/1 -> BCTire_Force_z/1  "L1"
  BCTire_Force_z/1 -> Tire_Force_z/1  "Tire_Force_z"

== system CRTsfun/VI-CarRealTime/Input_Bus/Inputs/Subsystem_Activation/Tire_Moment_x ==
  BCTire_Moment_x : BusCreator
  L1_def_val : Constant
  L2_def_val : Constant
  R1_def_val : Constant
  R2_def_val : Constant
  Tire_Moment_x : Outport
  wires:
  R2_def_val/1 -> BCTire_Moment_x/4  "R2"
  R1_def_val/1 -> BCTire_Moment_x/3  "R1"
  L2_def_val/1 -> BCTire_Moment_x/2  "L2"
  L1_def_val/1 -> BCTire_Moment_x/1  "L1"
  BCTire_Moment_x/1 -> Tire_Moment_x/1  "Tire_Moment_x"

== system CRTsfun/VI-CarRealTime/Input_Bus/Inputs/Subsystem_Activation/Tire_Moment_y ==
  BCTire_Moment_y : BusCreator
  L1_def_val : Constant
  L2_def_val : Constant
  R1_def_val : Constant
  R2_def_val : Constant
  Tire_Moment_y : Outport
  wires:
  R2_def_val/1 -> BCTire_Moment_y/4  "R2"
  R1_def_val/1 -> BCTire_Moment_y/3  "R1"
  L2_def_val/1 -> BCTire_Moment_y/2  "L2"
  L1_def_val/1 -> BCTire_Moment_y/1  "L1"
  BCTire_Moment_y/1 -> Tire_Moment_y/1  "Tire_Moment_y"

== system CRTsfun/VI-CarRealTime/Input_Bus/Inputs/Subsystem_Activation/Tire_Moment_z ==
  BCTire_Moment_z : BusCreator
  L1_def_val : Constant
  L2_def_val : Constant
  R1_def_val : Constant
  R2_def_val : Constant
  Tire_Moment_z : Outport
  wires:
  R2_def_val/1 -> BCTire_Moment_z/4  "R2"
  R1_def_val/1 -> BCTire_Moment_z/3  "R1"
  L2_def_val/1 -> BCTire_Moment_z/2  "L2"
  L1_def_val/1 -> BCTire_Moment_z/1  "L1"
  BCTire_Moment_z/1 -> Tire_Moment_z/1  "Tire_Moment_z"

== system CRTsfun/VI-CarRealTime/Input_Bus/Inputs/Third_Element/Damper_activity_flag ==
  BCDamper_activity_flag : BusCreator  Inputs=2
  front_def_val : Constant
  rear_def_val : Constant
  Damper_activity_flag : Outport
  wires:
  rear_def_val/1 -> BCDamper_activity_flag/2  "rear"
  front_def_val/1 -> BCDamper_activity_flag/1  "front"
  BCDamper_activity_flag/1 -> Damper_activity_flag/1  "Damper_activity_flag"

== system CRTsfun/VI-CarRealTime/Input_Bus/Inputs/Third_Element/Damper_force ==
  BCDamper_force : BusCreator  Inputs=2
  front_def_val : Constant  Value=0
  rear_def_val : Constant  Value=0
  Damper_force : Outport
  wires:
  rear_def_val/1 -> BCDamper_force/2  "rear"
  front_def_val/1 -> BCDamper_force/1  "front"
  BCDamper_force/1 -> Damper_force/1  "Damper_force"

== system CRTsfun/VI-CarRealTime/Input_Bus/Inputs/Third_Element/Spring ==
  BCSpring : BusCreator  Inputs=2
  front_def_val : Constant  Value=0
  rear_def_val : Constant  Value=0
  Spring : Outport
  wires:
  rear_def_val/1 -> BCSpring/2  "rear"
  front_def_val/1 -> BCSpring/1  "front"
  BCSpring/1 -> Spring/1  "Spring"

== system CRTsfun/VI-CarRealTime/Input_Bus/Inputs/Third_Element/Spring_activity_flag ==
  BCSpring_activity_flag : BusCreator  Inputs=2
  front_def_val : Constant
  rear_def_val : Constant
  Spring_activity_flag : Outport
  wires:
  rear_def_val/1 -> BCSpring_activity_flag/2  "rear"
  front_def_val/1 -> BCSpring_activity_flag/1  "front"
  BCSpring_activity_flag/1 -> Spring_activity_flag/1  "Spring_activity_flag"

== system CRTsfun/VI-CarRealTime/Input_Bus/Inputs/Tire_Force/Fx ==
  BCFx : BusCreator
  L1_def_val : Constant  Value=0
  L2_def_val : Constant  Value=0
  R1_def_val : Constant  Value=0
  R2_def_val : Constant  Value=0
  Fx : Outport
  wires:
  R2_def_val/1 -> BCFx/4  "R2"
  R1_def_val/1 -> BCFx/3  "R1"
  L2_def_val/1 -> BCFx/2  "L2"
  L1_def_val/1 -> BCFx/1  "L1"
  BCFx/1 -> Fx/1  "Fx"

== system CRTsfun/VI-CarRealTime/Input_Bus/Inputs/Tire_Force/Fy ==
  BCFy : BusCreator
  L1_def_val : Constant  Value=0
  L2_def_val : Constant  Value=0
  R1_def_val : Constant  Value=0
  R2_def_val : Constant  Value=0
  Fy : Outport
  wires:
  R2_def_val/1 -> BCFy/4  "R2"
  R1_def_val/1 -> BCFy/3  "R1"
  L2_def_val/1 -> BCFy/2  "L2"
  L1_def_val/1 -> BCFy/1  "L1"
  BCFy/1 -> Fy/1  "Fy"

== system CRTsfun/VI-CarRealTime/Input_Bus/Inputs/Tire_Force/Fz ==
  BCFz : BusCreator
  L1_def_val : Constant  Value=0
  L2_def_val : Constant  Value=0
  R1_def_val : Constant  Value=0
  R2_def_val : Constant  Value=0
  Fz : Outport
  wires:
  R2_def_val/1 -> BCFz/4  "R2"
  R1_def_val/1 -> BCFz/3  "R1"
  L2_def_val/1 -> BCFz/2  "L2"
  L1_def_val/1 -> BCFz/1  "L1"
  BCFz/1 -> Fz/1  "Fz"

== system CRTsfun/VI-CarRealTime/Input_Bus/Inputs/Tire_Moment/Mx ==
  BCMx : BusCreator
  L1_def_val : Constant  Value=0
  L2_def_val : Constant  Value=0
  R1_def_val : Constant  Value=0
  R2_def_val : Constant  Value=0
  Mx : Outport
  wires:
  R2_def_val/1 -> BCMx/4  "R2"
  R1_def_val/1 -> BCMx/3  "R1"
  L2_def_val/1 -> BCMx/2  "L2"
  L1_def_val/1 -> BCMx/1  "L1"
  BCMx/1 -> Mx/1  "Mx"

== system CRTsfun/VI-CarRealTime/Input_Bus/Inputs/Tire_Moment/My ==
  BCMy : BusCreator
  L1_def_val : Constant  Value=0
  L2_def_val : Constant  Value=0
  R1_def_val : Constant  Value=0
  R2_def_val : Constant  Value=0
  My : Outport
  wires:
  R2_def_val/1 -> BCMy/4  "R2"
  R1_def_val/1 -> BCMy/3  "R1"
  L2_def_val/1 -> BCMy/2  "L2"
  L1_def_val/1 -> BCMy/1  "L1"
  BCMy/1 -> My/1  "My"

== system CRTsfun/VI-CarRealTime/Input_Bus/Inputs/Tire_Moment/Mz ==
  BCMz : BusCreator
  L1_def_val : Constant  Value=0
  L2_def_val : Constant  Value=0
  R1_def_val : Constant  Value=0
  R2_def_val : Constant  Value=0
  Mz : Outport
  wires:
  R2_def_val/1 -> BCMz/4  "R2"
  R1_def_val/1 -> BCMz/3  "R1"
  L2_def_val/1 -> BCMz/2  "L2"
  L1_def_val/1 -> BCMz/1  "L1"
  BCMz/1 -> Mz/1  "Mz"

== system CRTsfun/VI-CarRealTime/Input_Bus/Inputs/Wheel_driving/moment ==
  BCmoment : BusCreator
  L1_def_val : Constant  Value=0
  L2_def_val : Constant  Value=0
  R1_def_val : Constant  Value=0
  R2_def_val : Constant  Value=0
  moment : Outport
  wires:
  R2_def_val/1 -> BCmoment/4  "R2"
  R1_def_val/1 -> BCmoment/3  "R1"
  L2_def_val/1 -> BCmoment/2  "L2"
  L1_def_val/1 -> BCmoment/1  "L1"
  BCmoment/1 -> moment/1  "moment"
